simulink model "rotor_resistance_control"  (R2014b)
settings: Solver=ode23tb  StartTime=0.0  StopTime=10.0  MaxStep=1e-4  RelTol=1e-3
libraries: powerlib x15
settings Model: Creator=Amr Saleh  LastModifiedBy=Amr Saleh

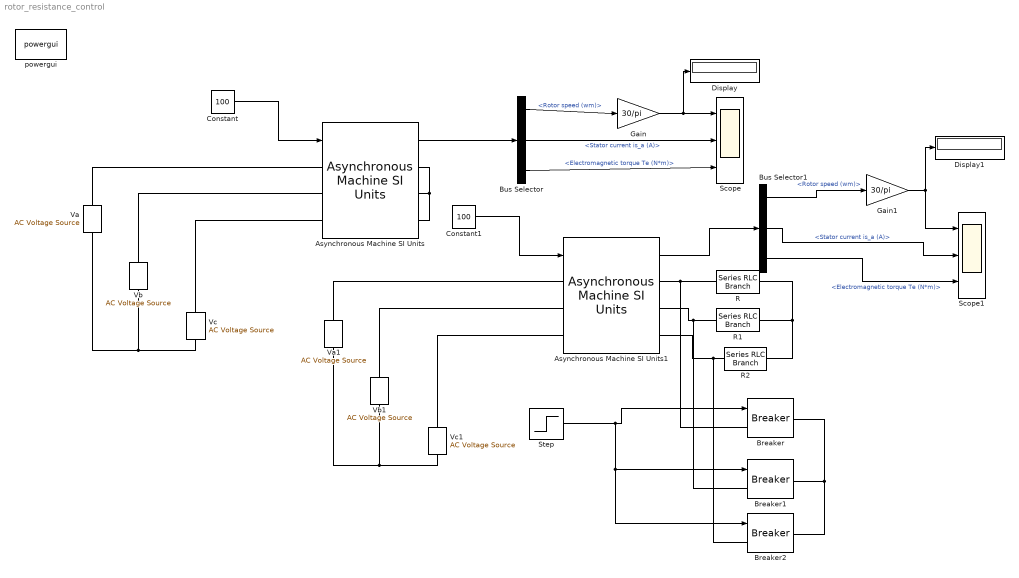
== system rotor_resistance_control ==
  Asynchronous Machine SI Units : powerlib/Machines/Asynchronous Machine SI Units  PresetModel=No  MechanicalLoad=Torque Tm  ShowDetailedParameters=on  RotorType=Wound  ReferenceFrame=Rotor  Units=SI  MeasurementBus=off  NominalParameters=[3.73e+04 460 50]  Stator=[0.09961 0.000867]  Rotor=[0.05837 0.000867]  Cage1=[ 0.022 0.226/377]  Cage2=[ 0.022 0.226/377]  Lm=0.03039  Mechanical=[0.4 0.02187 2]  PolePairs=2  InitialConditions=[1 0 0 0 0 0 0 0]  SimulateSaturation=off  Saturation=[14.03593122, 27.81365428, 53.79336849, 72.68890987, 97.98006896, 148.6815601, 215.7428561, 302.9841135, 420.4778367 ; 230, 322, 414, 460, 506, 552, 598, 644, 690]  LoadFlowParameters=1492000  TsPowergui=0  TsBlock=-1  IterativeModel=Trapezoidal non iterative  Pmec=0
  Asynchronous Machine SI Units1 : powerlib/Machines/Asynchronous Machine SI Units  PresetModel=No  MechanicalLoad=Torque Tm  ShowDetailedParameters=on  RotorType=Wound  ReferenceFrame=Rotor  Units=SI  MeasurementBus=off  NominalParameters=[3.73e+04 460 50]  Stator=[0.09961 0.000867]  Rotor=[0.05837 0.000867]  Cage1=[ 0.022 0.226/377]  Cage2=[ 0.022 0.226/377]  Lm=0.03039  Mechanical=[0.4 0.02187 2]  PolePairs=2  InitialConditions=[1 0 0 0 0 0 0 0]  SimulateSaturation=off  Saturation=[14.03593122, 27.81365428, 53.79336849, 72.68890987, 97.98006896, 148.6815601, 215.7428561, 302.9841135, 420.4778367 ; 230, 322, 414, 460, 506, 552, 598, 644, 690]  LoadFlowParameters=1492000  TsPowergui=0  TsBlock=-1  IterativeModel=Trapezoidal non iterative  Pmec=0
  Breaker : powerlib/Elements/Breaker  InitialState=0  SwitchingTimes="[1/60  5/60]"  External=on  BreakerResistance=0.01  SnubberResistance=1e6  SnubberCapacitance=inf  Measurements=None  MoreParameters=on  NoBreakLoop=off
  Breaker1 : powerlib/Elements/Breaker  InitialState=0  SwitchingTimes="[1/60  5/60]"  External=on  BreakerResistance=0.01  SnubberResistance=1e6  SnubberCapacitance=inf  Measurements=None  MoreParameters=on  NoBreakLoop=off
  Breaker2 : powerlib/Elements/Breaker  InitialState=0  SwitchingTimes="[1/60  5/60]"  External=on  BreakerResistance=0.01  SnubberResistance=1e6  SnubberCapacitance=inf  Measurements=None  MoreParameters=on  NoBreakLoop=off
  Bus Selector : BusSelector  OutputSignals=Mechanical.Rotor speed (wm),Stator measurements.Stator current is_a (A),Mechanical.Electromagnetic torque Te (N*m)
  Bus Selector1 : BusSelector  OutputSignals=Mechanical.Rotor speed (wm),Stator measurements.Stator current is_a (A),Mechanical.Electromagnetic torque Te (N*m)
  Constant : Constant  Value=100
  Constant1 : Constant  Value=100
  Display : Display
  Display1 : Display
  Gain : Gain  Gain=30/pi
  Gain1 : Gain  Gain=30/pi
  R : powerlib/Elements/Series RLC Branch  LConnTagsString=__new0  RConnTagsString=__new0  BranchType=R  Resistance=0.5  Inductance=1e-3  SetiL0=off  InitialCurrent=0  Capacitance=1e-6  Setx0=off  InitialVoltage=0  Measurements=None
  R1 : powerlib/Elements/Series RLC Branch  LConnTagsString=__new0  RConnTagsString=__new0  BranchType=R  Resistance=0.5  Inductance=1e-3  SetiL0=off  InitialCurrent=0  Capacitance=1e-6  Setx0=off  InitialVoltage=0  Measurements=None
  R2 : powerlib/Elements/Series RLC Branch  LConnTagsString=__new0  RConnTagsString=__new0  BranchType=R  Resistance=0.5  Inductance=1e-3  SetiL0=off  InitialCurrent=0  Capacitance=1e-6  Setx0=off  InitialVoltage=0  Measurements=None
  Scope : Scope  NumInputPorts=3
      settings: YMin=-5~-5~-5  YMax=5~5~5
  Scope1 : Scope  NumInputPorts=3
      settings: YMin=-5~-5~-5  YMax=5~5~5
  Step : Step  Time=0.25  SampleTime=0
  Va : powerlib/Electrical Sources/AC Voltage Source  Amplitude=376  Phase=0  Frequency=50  SampleTime=0  Measurements=None
  Va1 : powerlib/Electrical Sources/AC Voltage Source  Amplitude=376  Phase=0  Frequency=50  SampleTime=0  Measurements=None
  Vb : powerlib/Electrical Sources/AC Voltage Source  Amplitude=376  Phase=-120  Frequency=50  SampleTime=0  Measurements=None
  Vb1 : powerlib/Electrical Sources/AC Voltage Source  Amplitude=376  Phase=-120  Frequency=50  SampleTime=0  Measurements=None
  Vc : powerlib/Electrical Sources/AC Voltage Source  Amplitude=376  Phase=120  Frequency=50  SampleTime=0  Measurements=None
  Vc1 : powerlib/Electrical Sources/AC Voltage Source  Amplitude=376  Phase=120  Frequency=50  SampleTime=0  Measurements=None
  powergui : powerlib/powergui  Priority=1  SimulationMode=Continuous  SolverType=Tustin/Backward Euler (TBE)  SampleTime=50e-6  frequency=60  SPID=off  DisableSnubberDevices=off  DisableRonSwitches=off  DisableVfSwitches=off  SwTol=0  DisplayEquations=off  Interpol=off  methode=off  Ts=100  frequencyindice=50  Pbase=100e6  ErrMax=1e-4  Iterations=50  UnitsV=kV  UnitsW=MW  FunctionMessages=off  echomessages=off  HookPort=off  EnableUseOfTLC=off  x0status=blocks  RestoreLinks=warning  ResistiveCurrentMeasurement=off  Frange=[0:2:500]  Ylog=off  Xlog=on  ShowGrid=off  save=off  variable=ZData  structure=0  ZoomFFT=off  StartTime=0.0  cycles=1  DisplayStyle=1  fundamental=60  FreqAxis=off  MaxFrequency=1000  frequencyindicesteady=1  RmsSteady=1  display=off
  wires:
  Constant/1 -> Asynchronous Machine SI Units/1
  Asynchronous Machine SI Units/1 -> Bus Selector/1
  Bus Selector/1 -> Gain/1  "<Rotor speed (wm)>"
  Bus Selector/2 -> Scope/2  "<Stator current is_a (A)>"
  Bus Selector/3 -> Scope/3  "<Electromagnetic torque Te (N*m)>"
  Gain/1 -> Display/1, Scope/1
  Constant1/1 -> Asynchronous Machine SI Units1/1
  Asynchronous Machine SI Units1/1 -> Bus Selector1/1
  Bus Selector1/1 -> Gain1/1  "<Rotor speed (wm)>"
  Bus Selector1/2 -> Scope1/2  "<Stator current is_a (A)>"
  Bus Selector1/3 -> Scope1/3  "<Electromagnetic torque Te (N*m)>"
  Gain1/1 -> Scope1/1, Display1/1
  Step/1 -> Breaker2/1, Breaker1/1, Breaker/1
  connections:
  Asynchronous Machine SI Units/RConn1 -- Asynchronous Machine SI Units/RConn2 -- Asynchronous Machine SI Units/RConn3
  Va/RConn1 -- Asynchronous Machine SI Units/LConn1
  Vb/RConn1 -- Asynchronous Machine SI Units/LConn2
  Vc/RConn1 -- Asynchronous Machine SI Units/LConn3
  Vc/LConn1 -- Vb/LConn1 -- Va/LConn1
  Vb1/LConn1 -- Vc1/LConn1 -- Va1/LConn1
  Vc1/RConn1 -- Asynchronous Machine SI Units1/LConn3
  Va1/RConn1 -- Asynchronous Machine SI Units1/LConn1
  Vb1/RConn1 -- Asynchronous Machine SI Units1/LConn2
  R/LConn1 -- Breaker/LConn1 -- Asynchronous Machine SI Units1/RConn1
  R1/LConn1 -- Breaker1/LConn1 -- Asynchronous Machine SI Units1/RConn2
  R2/LConn1 -- Breaker2/LConn1 -- Asynchronous Machine SI Units1/RConn3
  R/RConn1 -- R1/RConn1 -- R2/RConn1
  Breaker/RConn1 -- Breaker1/RConn1 -- Breaker2/RConn1
